simulink model "partSeven"  (R2021b)
settings: Solver=VariableStepAuto  StartTime=0.0  StopTime=10  RelTol=1e-3
libraries: simulink x2
settings Model: Creator=ericp  LastModifiedBy=ericp

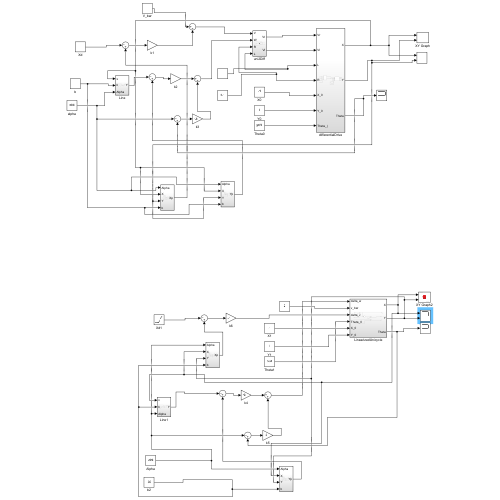
[thumbnail: Simulink's stored preview of the top-level diagram]
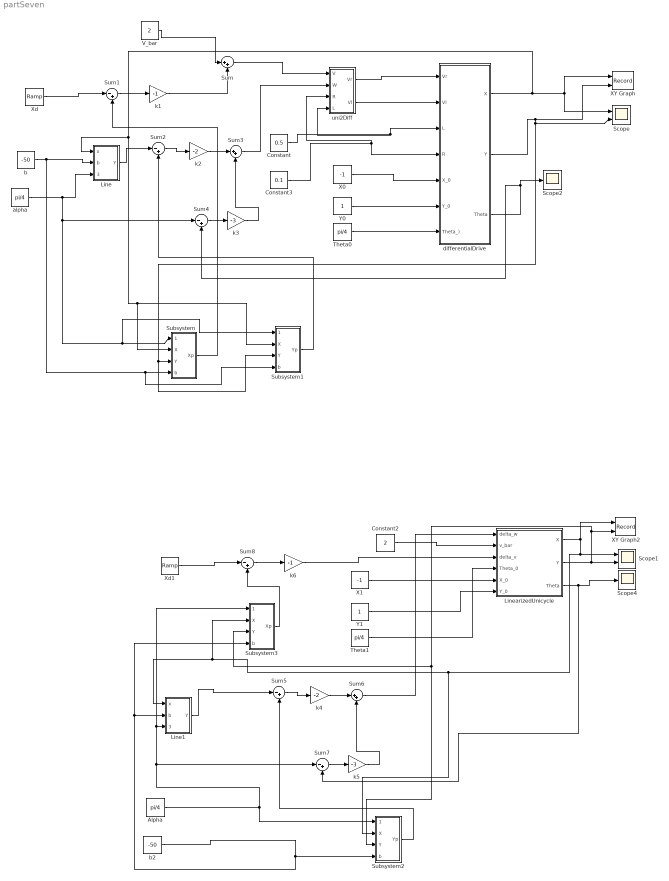
== system partSeven ==
  Alpha : Constant  Value=pi/4
  Constant : Constant  Value=0.5
  Constant2 : Constant  Value=2
  Constant3 : Constant  Value=0.1
  Line : Subsystem
  Line1 : Subsystem
  LinearizedUnicycle : Subsystem
  Scope : Scope  NumInputPorts=2
  Scope1 : Scope  NumInputPorts=2
  Scope2 : Scope
  Scope4 : Scope
  Subsystem : Subsystem
  Subsystem1 : Subsystem
  Subsystem2 : Subsystem
  Subsystem3 : Subsystem
  Sum : Sum  Inputs=|++
  Sum{1..2,4..5,7..8} (6 alike) : Sum  Inputs=|-+
  Sum3 : Sum  Inputs=|++
  Sum6 : Sum  Inputs=|++
  Theta0 : Constant  Value=pi/4
  Theta1 : Constant  Value=pi/4
  V_bar : Constant  Value=2
  X0 : Constant  Value=-1
  X1 : Constant  Value=-1
  XY Graph : Record  FileSettingsInternal="{\"entries\":[{\"content\":{\"excelSettings\":{\"content\":{},\"type\":\"Streamout.ExcelSettings\"}},\"type\":\"Streamout.FileSettingStorage\",\"uuid\":\"3fa76106-a2ad-4ab3-86b9-e47068223577\"}],\"packageUris\":[\"http://schema.mathworks.com/mf0/streamout_blocks/R2020a\"],\"version\":\"1.0\"}"  Layout=[1 1]  SignalsInternal="{\"entries\":[{\"content\":{\"signals\":[{\"content\":{\"blockPath\":[\"part7/XY Graph\"],\"channel\":[],\"dimensions\":[1],\"domain\":\"part7/XY Graph\",\"lineColor\":\"#77ac30\",\"plots\":[1],\"port\":1,\"sid\":[\"\"],\"signalID\":3570,\"signalName\":\"differentialDrive:1\"},\"type\":\"RecordBlkView.Signal\",\"uuid\":\"0ac4baac-7a82-4ac9-a222-7ae5cd6d6832\"},{\"content\":{\"blockPath\":[\"part7/XY Graph\"],\"channel\":[],\"dimensions\":[1],\"domain\":\"part7/XY Graph\",\"lineColor\":\"#4dbeee\",\"plots\":[1],\"port\":2,\"sid\":[\"\"],\"signalID\":3574,\"signalName\":\"differentialDrive:2\"},\"type\":\"RecordBlkView.Signal\",\"uuid\":\"a4149277-f40e-45f2-ba70-0db66da1e906\"}]},\"type\":\"RecordBlkView.InputSignals\",\"uuid\":\"0bb04f89-936d-44ab-88d7-b5f2b34e02ec\"}],\"packageUris\":[\"http://schema.mathworks.com/mf0/streamout_blocks/R2020a\"],\"version\":\"1.0\"}"  VisualizationBindings="{\"xyplotplugin\":{\"info\":[{\"series\":[{\"bindingParametersList\":[{\"parameter\":\"Y-Axis\",\"signalID\":3574,\"signalName\":\"differentialDrive:2\"},{\"parameter\":\"X-Axis\",\"signalID\":3570,\"signalName\":\"differentialDrive:1\"}],\"seriesID\":522}],\"subplotID\":1}]}}"  CompatibilityTag=XY
  XY Graph2 : Record  FileSettingsInternal="{\"entries\":[{\"content\":{\"excelSettings\":{\"content\":{},\"type\":\"Streamout.ExcelSettings\"}},\"type\":\"Streamout.FileSettingStorage\",\"uuid\":\"28221481-41f6-45ca-9cbf-c59e26c50b4a\"}],\"packageUris\":[\"http://schema.mathworks.com/mf0/streamout_blocks/R2020a\"],\"version\":\"1.0\"}"  Layout=[1 1]  SignalsInternal="{\"entries\":[{\"content\":{\"signals\":[{\"content\":{\"blockPath\":[\"part7/XY Graph2\"],\"channel\":[],\"dimensions\":[1],\"domain\":\"part7/XY Graph2\",\"lineColor\":\"#a2142f\",\"plots\":[1],\"port\":1,\"sid\":[\"\"],\"signalID\":3562,\"signalName\":\"LinearizedUnicycle:1\"},\"type\":\"RecordBlkView.Signal\",\"uuid\":\"5c1d0093-739a-41fe-9446-775ddbbc40c1\"},{\"content\":{\"blockPath\":[\"part7/XY Graph2\"],\"channel\":[],\"dimensions\":[1],\"domain\":\"part7/XY Graph2\",\"lineColor\":\"#139fff\",\"plots\":[1],\"port\":2,\"sid\":[\"\"],\"signalID\":3566,\"signalName\":\"LinearizedUnicycle:2\"},\"type\":\"RecordBlkView.Signal\",\"uuid\":\"89f75605-0ec3-4324-ae99-3ea2d6bff75e\"}]},\"type\":\"RecordBlkView.InputSignals\",\"uuid\":\"af6b47c5-a190-4ece-b1b0-1f9f54fadfc9\"}],\"packageUris\":[\"http://schema.mathworks.com/mf0/streamout_blocks/R2020a\"],\"version\":\"1.0\"}"  VisualizationBindings="{\"xyplotplugin\":{\"info\":[{\"series\":[{\"bindingParametersList\":[{\"parameter\":\"Y-Axis\",\"signalID\":3566,\"signalName\":\"LinearizedUnicycle:2\"},{\"parameter\":\"X-Axis\",\"signalID\":3562,\"signalName\":\"LinearizedUnicycle:1\"}],\"seriesID\":4905}],\"subplotID\":1}]}}"  CompatibilityTag=XY
  Xd : simulink/Sources/Ramp  slope=1  start=0  InitialOutput=0
  Xd1 : simulink/Sources/Ramp  slope=1  start=0  InitialOutput=0
  Y0 : Constant
  Y1 : Constant
  alpha : Constant  Value=pi/4
  b : Constant  Value=-50
  b2 : Constant  Value=-50
  differentialDrive : Subsystem
  k1 : Gain  Gain=-1
  k2 : Gain  Gain=-2
  k3 : Gain  Gain=-3
  k4 : Gain  Gain=-2
  k5 : Gain  Gain=-3
  k6 : Gain  Gain=-1
  uni2Diff : Subsystem
  wires:
  Xd/1 -> Sum1/1
  Theta0/1 -> differentialDrive/7(Theta_))
  Y0/1 -> differentialDrive/6(Y_0)
  k2/1 -> Sum3/1
  Sum4/1 -> k3/1
  Sum3/1 -> uni2Diff/2(W)
  k1/1 -> Sum/2
  V_bar/1 -> Sum/1
  X0/1 -> differentialDrive/5(X_0)
  Sum2/1 -> k2/1
  Constant3/1 -> differentialDrive/4(R), uni2Diff/3(R)
  k3/1 -> Sum3/2
  differentialDrive/1(X) -> Line/1(x), Subsystem1/2(X), Subsystem/2(X), XY Graph/1, Scope/1
  uni2Diff/1(Vr) -> differentialDrive/1(Vr)
  Constant/1 -> uni2Diff/4(L), differentialDrive/3(L)
  differentialDrive/2(Y) -> XY Graph/2, Subsystem1/3(Y), Subsystem/3(Y), Scope/2
  uni2Diff/2(Vl) -> differentialDrive/2(Vl)
  Sum1/1 -> k1/1
  differentialDrive/3(Theta) -> Scope2/1, Sum4/2
  Sum/1 -> uni2Diff/1(V)
  Line/1(Y) -> Sum2/1
  b/1 -> Subsystem1/4("b "), Subsystem/4("b "), Line/2(b)
  alpha/1 -> Line/3(Alpha), Subsystem1/1(Alpha), Subsystem/1(Alpha), Sum4/1
  Subsystem/1(Xp) -> Sum1/2
  Subsystem1/1(Yp) -> Sum2/2
  LinearizedUnicycle/2(Y) -> Subsystem3/3(Y), Subsystem2/3(Y), XY Graph2/2, Scope1/2
  Sum7/1 -> k5/1
  Sum8/1 -> k6/1
  Xd1/1 -> Sum8/1
  LinearizedUnicycle/1(X) -> XY Graph2/1, Scope1/1, Subsystem3/2(X), Line1/1(x), Subsystem2/2(X)
  k5/1 -> Sum6/2
  k4/1 -> Sum6/1
  k6/1 -> LinearizedUnicycle/3(delta_v)
  Y1/1 -> LinearizedUnicycle/6(Y_0)
  LinearizedUnicycle/3(Theta) -> Sum7/2, Scope4/1
  Constant2/1 -> LinearizedUnicycle/2(v_bar)
  Sum5/1 -> k4/1
  Sum6/1 -> LinearizedUnicycle/1(delta_w)
  Theta1/1 -> LinearizedUnicycle/4(Theta_0)
  X1/1 -> LinearizedUnicycle/5(X_0)
  Subsystem2/1(Yp) -> Sum5/2
  Alpha/1 -> Subsystem2/1(Alpha), Subsystem3/1(Alpha), Line1/3(Alpha), Sum7/1
  b2/1 -> Subsystem3/4("b "), Line1/2(b), Subsystem2/4("b ")
  Line1/1(Y) -> Sum5/1
  Subsystem3/1(Xp) -> Sum8/2

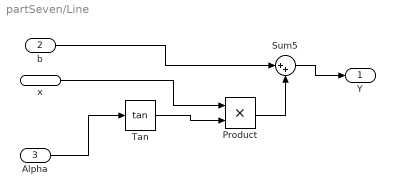
== system partSeven/Line ==
  x : Inport
  b : Inport  Port=2
  Alpha : Inport  Port=3
  Product : Product
  Sum5 : Sum  Inputs=|++
  Tan : Trigonometry  Operator=tan
  Y : Outport
  wires:
  Alpha/1 -> Tan/1
  Sum5/1 -> Y/1
  x/1 -> Product/1
  Tan/1 -> Product/2
  Product/1 -> Sum5/2
  b/1 -> Sum5/1

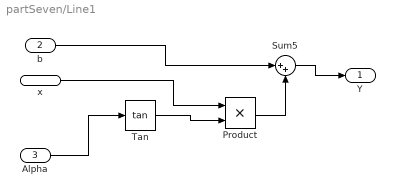
== system partSeven/Line1 ==
  x : Inport
  b : Inport  Port=2
  Alpha : Inport  Port=3
  Product : Product
  Sum5 : Sum  Inputs=|++
  Tan : Trigonometry  Operator=tan
  Y : Outport
  wires:
  Alpha/1 -> Tan/1
  Sum5/1 -> Y/1
  x/1 -> Product/1
  Tan/1 -> Product/2
  Product/1 -> Sum5/2
  b/1 -> Sum5/1

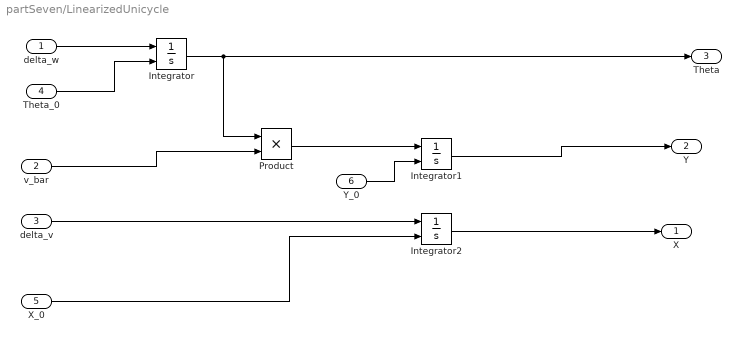
== system partSeven/LinearizedUnicycle ==
  delta_w : Inport
  v_bar : Inport  Port=2
  delta_v : Inport  Port=3
  Theta_0 : Inport  Port=4
  X_0 : Inport  Port=5
  Y_0 : Inport  Port=6
  Integrator : Integrator  InitialConditionSource=external
  Integrator1 : Integrator  InitialConditionSource=external
  Integrator2 : Integrator  InitialConditionSource=external
  Product : Product
  X : Outport
  Y : Outport  Port=2
  Theta : Outport  Port=3
  wires:
  Integrator/1 -> Theta/1, Product/1
  Theta_0/1 -> Integrator/2
  v_bar/1 -> Product/2
  Product/1 -> Integrator1/1
  delta_w/1 -> Integrator/1
  X_0/1 -> Integrator2/2
  Integrator1/1 -> Y/1
  Y_0/1 -> Integrator1/2
  delta_v/1 -> Integrator2/1
  Integrator2/1 -> X/1

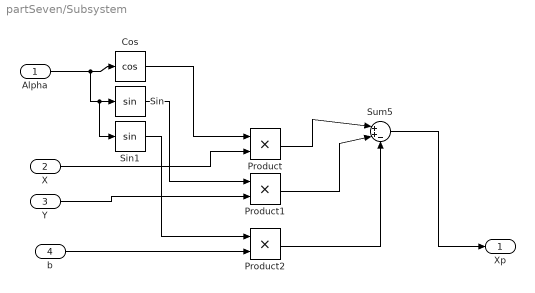
== system partSeven/Subsystem ==
  Alpha : Inport
  X : Inport  Port=2
  Y : Inport  Port=3
  "b " : Inport  Port=4
  Cos : Trigonometry  Operator=cos
  Product : Product
  Product1 : Product
  Product2 : Product
  Sin : Trigonometry
  Sin1 : Trigonometry
  Sum5 : Sum  Inputs=|++-
  Xp : Outport
  wires:
  X/1 -> Product/2
  Alpha/1 -> Sin1/1, Sin/1, Cos/1
  Sin/1 -> Product1/1
  Product2/1 -> Sum5/3
  Product/1 -> Sum5/1
  Cos/1 -> Product/1
  Product1/1 -> Sum5/2
  Sin1/1 -> Product2/1
  Y/1 -> Product1/2
  "b "/1 -> Product2/2
  Sum5/1 -> Xp/1

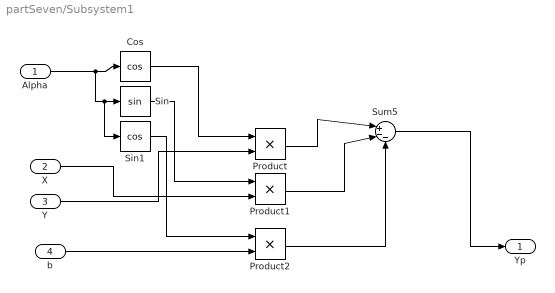
== system partSeven/Subsystem1 ==
  Alpha : Inport
  X : Inport  Port=2
  Y : Inport  Port=3
  "b " : Inport  Port=4
  Cos : Trigonometry  Operator=cos
  Product : Product
  Product1 : Product
  Product2 : Product
  Sin : Trigonometry
  Sin1 : Trigonometry  Operator=cos
  Sum5 : Sum  Inputs=|+--
  Yp : Outport
  wires:
  Alpha/1 -> Sin1/1, Sin/1, Cos/1
  X/1 -> Product1/2
  Product1/1 -> Sum5/2
  Y/1 -> Product/2
  Sum5/1 -> Yp/1
  "b "/1 -> Product2/2
  Product/1 -> Sum5/1
  Product2/1 -> Sum5/3
  Sin/1 -> Product1/1
  Sin1/1 -> Product2/1
  Cos/1 -> Product/1

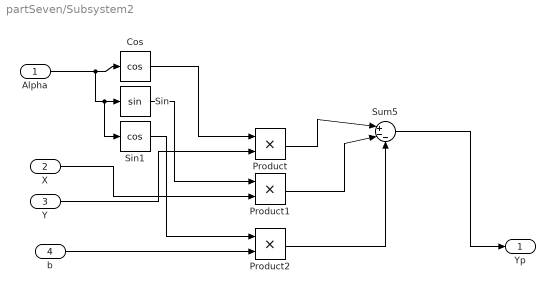
== system partSeven/Subsystem2 ==
  Alpha : Inport
  X : Inport  Port=2
  Y : Inport  Port=3
  "b " : Inport  Port=4
  Cos : Trigonometry  Operator=cos
  Product : Product
  Product1 : Product
  Product2 : Product
  Sin : Trigonometry
  Sin1 : Trigonometry  Operator=cos
  Sum5 : Sum  Inputs=|+--
  Yp : Outport
  wires:
  Alpha/1 -> Sin1/1, Sin/1, Cos/1
  X/1 -> Product1/2
  Product1/1 -> Sum5/2
  Y/1 -> Product/2
  Sum5/1 -> Yp/1
  "b "/1 -> Product2/2
  Product/1 -> Sum5/1
  Product2/1 -> Sum5/3
  Sin/1 -> Product1/1
  Sin1/1 -> Product2/1
  Cos/1 -> Product/1

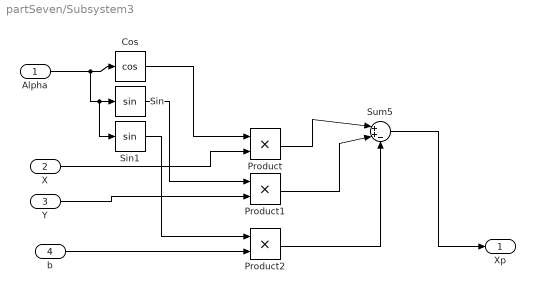
== system partSeven/Subsystem3 ==
  Alpha : Inport
  X : Inport  Port=2
  Y : Inport  Port=3
  "b " : Inport  Port=4
  Cos : Trigonometry  Operator=cos
  Product : Product
  Product1 : Product
  Product2 : Product
  Sin : Trigonometry
  Sin1 : Trigonometry
  Sum5 : Sum  Inputs=|++-
  Xp : Outport
  wires:
  X/1 -> Product/2
  Alpha/1 -> Sin1/1, Sin/1, Cos/1
  Sin/1 -> Product1/1
  Product2/1 -> Sum5/3
  Product/1 -> Sum5/1
  Cos/1 -> Product/1
  Product1/1 -> Sum5/2
  Sin1/1 -> Product2/1
  Y/1 -> Product1/2
  "b "/1 -> Product2/2
  Sum5/1 -> Xp/1

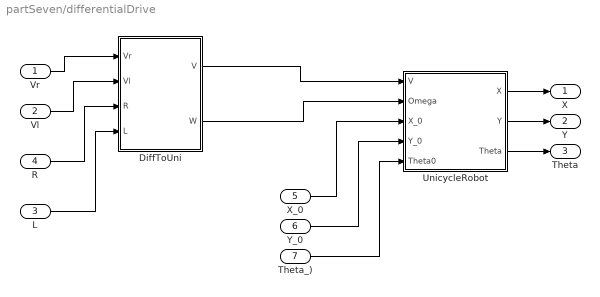
== system partSeven/differentialDrive ==
  Vr : Inport
  Vl : Inport  Port=2
  L : Inport  Port=3
  R : Inport  Port=4
  X_0 : Inport  Port=5
  Y_0 : Inport  Port=6
  Theta_) : Inport  Port=7
  DiffToUni : Subsystem
  UnicycleRobot : Subsystem
  X : Outport
  Y : Outport  Port=2
  Theta : Outport  Port=3
  wires:
  Y_0/1 -> UnicycleRobot/4(Y_0)
  UnicycleRobot/3(Theta) -> Theta/1
  UnicycleRobot/1(X) -> X/1
  UnicycleRobot/2(Y) -> Y/1
  DiffToUni/1(V) -> UnicycleRobot/1(V)
  Theta_)/1 -> UnicycleRobot/5(Theta0)
  Vr/1 -> DiffToUni/1(Vr)
  DiffToUni/2(W) -> UnicycleRobot/2(Omega)
  R/1 -> DiffToUni/3(R)
  Vl/1 -> DiffToUni/2(Vl)
  L/1 -> DiffToUni/4(L)
  X_0/1 -> UnicycleRobot/3(X_0)

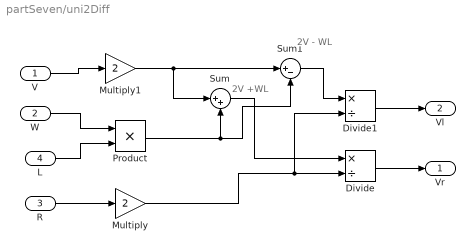
== system partSeven/uni2Diff ==
  note: 2V +WL
  note: 2V - WL
  V : Inport
  W : Inport  Port=2
  R : Inport  Port=3
  L : Inport  Port=4
  Divide : Product  Inputs=*/
  Divide1 : Product  Inputs=*/
  Multiply : Gain  Gain=2
  Multiply1 : Gain  Gain=2
  Product : Product
  Sum : Sum  Inputs=|++
  Sum1 : Sum  Inputs=|+-
  Vr : Outport
  Vl : Outport  Port=2
  wires:
  V/1 -> Multiply1/1
  Divide/1 -> Vr/1
  Sum1/1 -> Divide1/1
  Multiply/1 -> Divide1/2, Divide/2
  Divide1/1 -> Vl/1
  L/1 -> Product/2
  R/1 -> Multiply/1
  Multiply1/1 -> Sum1/1, Sum/1
  Sum/1 -> Divide/1
  Product/1 -> Sum1/2, Sum/2
  W/1 -> Product/1

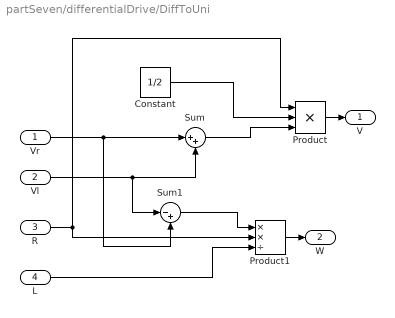
== system partSeven/differentialDrive/DiffToUni ==
  Vr : Inport
  Vl : Inport  Port=2
  R : Inport  Port=3
  L : Inport  Port=4
  Constant : Constant  Value=1/2
  Product : Product  Inputs=3
  Product1 : Product  Inputs=**/  InputSameDT=on
  Sum : Sum  Inputs=|++
  Sum1 : Sum  Inputs=|-+
  V : Outport
  W : Outport  Port=2
  wires:
  Vl/1 -> Sum1/1, Sum/2
  L/1 -> Product1/3
  Sum/1 -> Product/3
  Vr/1 -> Sum1/2, Sum/1
  R/1 -> Product1/2, Product/1
  Constant/1 -> Product/2
  Sum1/1 -> Product1/1
  Product/1 -> V/1
  Product1/1 -> W/1

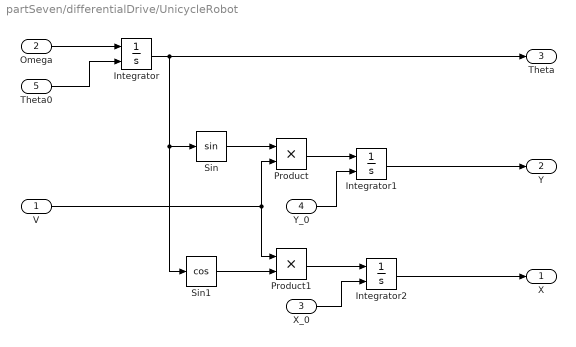
== system partSeven/differentialDrive/UnicycleRobot ==
  V : Inport
  Omega : Inport  Port=2
  X_0 : Inport  Port=3
  Y_0 : Inport  Port=4
  Theta0 : Inport  Port=5
  Integrator : Integrator  InitialConditionSource=external
  Integrator1 : Integrator  InitialConditionSource=external
  Integrator2 : Integrator  InitialConditionSource=external
  Product : Product
  Product1 : Product
  Sin : Trigonometry
  Sin1 : Trigonometry  Operator=cos
  X : Outport
  Y : Outport  Port=2
  Theta : Outport  Port=3
  wires:
  Sin1/1 -> Product1/2
  V/1 -> Product1/1, Product/2
  Integrator/1 -> Theta/1, Sin1/1, Sin/1
  Integrator2/1 -> X/1
  Sin/1 -> Product/1
  Theta0/1 -> Integrator/2
  Y_0/1 -> Integrator1/2
  Omega/1 -> Integrator/1
  X_0/1 -> Integrator2/2
  Integrator1/1 -> Y/1
  Product1/1 -> Integrator2/1
  Product/1 -> Integrator1/1
